simulink model "combined_models_v16"  (R2021a)
settings: Solver=VariableStepAuto  StartTime=0.0  StopTime=30  RelTol=1e-3
values from neighbouring files (symbols this model uses):
  r__s_st = r__s_stCG - r__t_tCG    [init_saildrone_dynamics_v5.m]    (also in moduleBasedModel_v7.m = cfg.r__s_st; systemVelocities.m = cfg.r__s_st)
  r__t_tAC = r__t_tCG    [init_saildrone_dynamics_v5.m]
  rho = 1025    [init_saildrone_dynamics_v5.m]    (also in moduleBasedModel_v7.m = cfg.rho; simplifiedModel_v8.m = cfg.rho)
  rho_air = 1.225    [init_saildrone_dynamics_v5.m]
undefined symbols (not defined in the file or in its folder): beta_V_w, cfg, delta_LOS, DiscIntNeverNeededParam, gamma_c, GWP, heading_controller_samplingtime, heading_rate_ref, K_b, K_d_heading, K_d_heading2, K_d_s, k_d_s, K_d_t, K_i_heading, K_i_heading2, K_i_s, k_i_s, K_i_t, K_p_heading, K_p_heading2, k_p_s, K_p_s, K_p_t, Ka_lin, keel, ObjectsPosition, omega_n_heading2, omega_n_s, q0, q_dot0, rudder, sail, sail_AOA_controller_samplingtime, sail_AOA_linearization_point, sail_AOA_saturation, sail_AOA_table, simulation_sampling_time, start_w_trans, tacking_minus, tacking_plus, tail, theta0, timeconstant_w, U_c, U_linearization_heading, U_w, U_w_step, v_current, v_wind, v_wind_unit, wn_ref_heading, wn_ref_t, xi0, zeta_ref_heading, zeta_ref_t
(part 1 of 3)
settings Model: Creator=jorge  LastModifiedBy=jorge

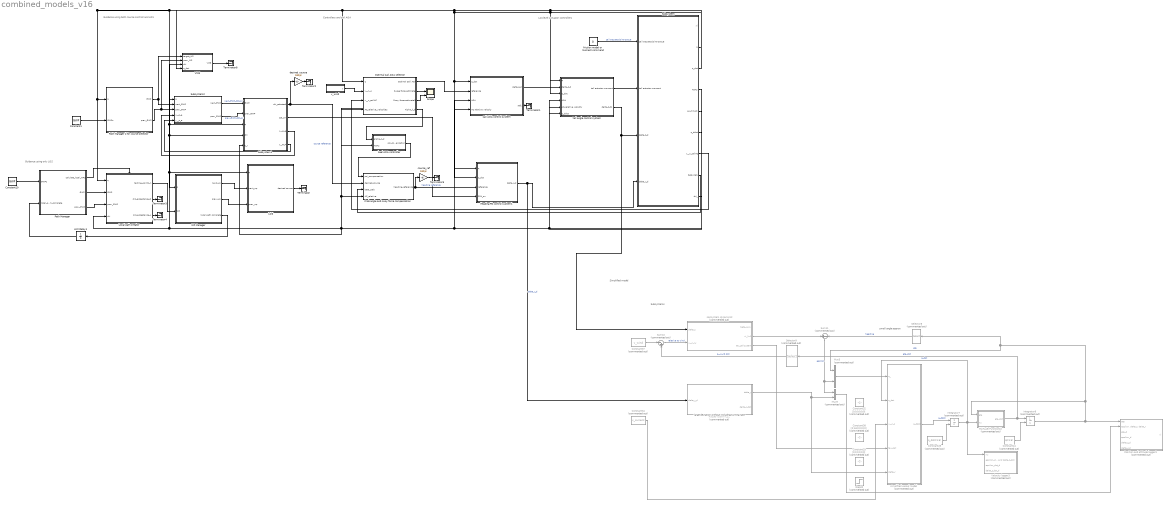
== system combined_models_v16 ==
  note: Guidance using only LOS
  note: Guidance using both course controll and LOS
  note: Controllers and sail AOA
  note: Lowlevel Actuator controllers
  note: Subsystems
  note: small angle approx
  note: large deviation without including turning rate
  note: Simplified model
  Constant1 : Constant  Value=GWP
  Constant10 : Constant  Value=GWP
  Constant24 : Constant  Commented=on  Value=q0(1:6)
  Constant25 : Constant  Commented=on  Value=q_dot0(1:6)
  Constant32 : Constant  Commented=on  Value=[0;0;0;0;0;0]
  Constant33 : Constant  Commented=on  Value=[0;0;0;0;0;0]
  Constant34 : Constant  Commented=on  Value=v_current
  Constant37 : Constant  Commented=on  Value=v_wind
  Constant38 : Constant  Commented=on  Value=[0;140;0;0;0;0]
  "Crab angle and sway force compensation " : MATLAB Function  TreatAsAtomicUnit=on
  Heading PD control system1 : Subsystem
  Integrator7 : Integrator  Commented=on  InitialConditionSource=external
  Integrator8 : Integrator  Commented=on  InitialConditionSource=external
  LOS : Subsystem
  Local path creator : Subsystem
  MATLAB Function10 : MATLAB Function  Commented=on  TreatAsAtomicUnit=on
  Mux3 : Mux  Commented=on  Inputs=2
  Mux9 : Mux  Commented=on  Inputs=3
  Optimal sail AOA selector : Subsystem
  Path Manager : Subsystem
  Path Manager 2 for course selector : Subsystem
  Position and attitude logger3 : Subsystem  Commented=on
  Rudder dyanmics2 : Subsystem  Commented=on
  Scope : Scope  NumInputPorts=2
  Selector8 : Selector  Commented=on  InputPortWidth=6  IndexOptions=Index vector (dialog)  Indices=[6]  OutputSizes=1
  Selector9 : Selector  Commented=on  InputPortWidth=6  IndexOptions=Index vector (dialog)  Indices="[1  2 3]"  OutputSizes=1
  Step20 : Step  Commented=on  After=-pi/4*1  SampleTime=0
  Subsystem : Subsystem
  Subsystem1 : Subsystem
  Subsystem2 : Subsystem
  Sum10 : Sum  Commented=on  Inputs=|-+
  Sum11 : Sum  Commented=on  Inputs=+-
  Terminator{,1..5,8} (7 alike) : Terminator
  Unit Delay1 : UnitDelay  SampleTime=-1  HasFrameUpgradeWarning=on
  VMG : MATLAB Function  TreatAsAtomicUnit=on
  Velocity logger3 : Subsystem  Commented=on
  WP Manager : Subsystem
  course_ref : Gain  Gain=180/pi
  desired_course : Gain  Gain=180/pi
  friction model or moment command : Constant  Value=0
  keel AOA controller : Subsystem
  sail AOA control system : Subsystem
  sailsystem dynamics2 : Subsystem  Commented=on
  simplified vessel model : MATLAB Function  Commented=on  TreatAsAtomicUnit=on
  tail angle control system : Subsystem
  v_wind : Subsystem
  wires:
  friction model or moment command/1 -> Subsystem/1(sail actuator/joint torque)  "sail actuator/joint torque"
  Subsystem/4(AOAs) -> tail angle control system/4(AOA), sail AOA control system/3(AOA), keel AOA controller/2(AOAs)
  Subsystem/3(q_dot) -> Heading PD control system1/2(q_dot), sail AOA control system/1(q_dot), VMG/4(q_dot), tail angle control system/3(q_dot)
  Subsystem/6(q_ddot) -> tail angle control system/6(q_ddot)
  tail angle control system/1(tail actuator moment) -> Subsystem/2(tail actuator moment)
  Subsystem/5(U_r_linkAC) -> tail angle control system/5(AC_relative velocity), sail AOA control system/4(AC relative velocity), Optimal sail AOA selector/4(AC_relative_velocities), "Crab angle and sway force compensation "/4(AC_relative), Subsystem1/5(U_r)
  Subsystem/7(v__n_sailAC) -> Optimal sail AOA selector/3(v__n_sailAC)
  Optimal sail AOA selector/2(Surge force estimate) -> Scope/1
  Optimal sail AOA selector/3(Sway force estimate1) -> Scope/2
  Subsystem/2(q) -> Heading PD control system1/1(q), Path Manager 2 for course selector/1(q), Local path creator/1(q), Subsystem2/1(q), Subsystem1/3(q), WP Manager/1(q), LOS/1(q), Optimal sail AOA selector/1(q), tail angle control system/1(q)
  sail AOA control system/2(ref1) -> Terminator1/1
  Constant24/1 -> Integrator8/2
  sailsystem dynamics2/3(tau_sailsystem) -> simplified vessel model/4(tau_sail)
  Constant25/1 -> Integrator7/2
  Rudder dyanmics2/1(delta_r) -> simplified vessel model/5(delta_r), Mux9/3
  Sum11/1 -> Mux3/2, Mux9/1  "epsilon"
  Integrator8/1 -> Selector8/1, Mux3/1, MATLAB Function10/1(eta), Position and attitude logger3/1(eta)  "eta"
  Constant34/1 -> simplified vessel model/3(v__n_c)
  Heading PD control system1/1(delta_r_d) -> Rudder dyanmics2/1(delta_r_d), Subsystem/4(delta_r_d)  "delta_r_d"
  Mux9/1 -> Position and attitude logger3/2("epsilon, delta_t, delta_r")
  Selector9/1 -> Sum10/2  "p__n_nb dot"
  simplified vessel model/1(q_ddot) -> Integrator7/1  "q_ddot"
  Sum10/1 -> sailsystem dynamics2/2(v__n_rw)  "relative to wind"
  Integrator7/1 -> Velocity logger3/1(nu), MATLAB Function10/2(nu), simplified vessel model/2(q_dot)  "q_dot"
  Selector8/1 -> Sum11/2  "heading"
  Constant37/1 -> Sum10/1
  sailsystem dynamics2/2(xi_lin1) -> Sum11/1
  MATLAB Function10/1(eta_dot) -> Selector9/1, Integrator8/1  "eta_dot"
  Mux3/1 -> simplified vessel model/1(q_)
  Optimal sail AOA selector/4(Alpha_k_d) -> keel AOA controller/1(alpha_k_d)
  Subsystem1/1(chi_selected) -> "Crab angle and sway force compensation "/2(desired_course), desired_course/1  "course reference"
  Subsystem/8(beta crab) -> "Crab angle and sway force compensation "/3(beta_crab)
  desired_course/1 -> Terminator2/1
  WP Manager/1(next_wp) -> LOS/2(next_wp)
  WP Manager/2(prev_wp) -> LOS/3(prev_wp)
  keel AOA controller/1(psi_compensation) -> "Crab angle and sway force compensation "/1(psi_compensation)
  WP Manager/3(local path complete) -> Unit Delay1/1
  Local path creator/2(circ_acceptance_R) -> Terminator3/1
  Local path creator/1(tacking_points_n) -> WP Manager/2(WP)
  Local path creator/3(circ_acceptance_L) -> Terminator4/1
  Subsystem/9(chi_) -> VMG/3(chi), Subsystem1/4(chi), Local path creator/4(chi)
  Path Manager/1(calulate_local_WPs) -> Local path creator/Enable
  Path Manager/3(prev_GWP) -> Local path creator/3(prev_GWP)
  Path Manager/2(GWP) -> Local path creator/2(GWP)
  Constant10/1 -> Path Manager/1(GWPs)
  Unit Delay1/1 -> Path Manager/2(local_path_complete)
  Constant1/1 -> Path Manager 2 for course selector/2(GWPs)
  Subsystem1/2(ssa_on) -> Heading PD control system1/4(SSA_on)
  Subsystem1/3(x__p_e) -> Subsystem2/4(x__p_e)
  Subsystem1/4(y__e_p) -> Subsystem2/5(y__p_e)
  Path Manager 2 for course selector/1(GWP) -> VMG/1(target_WP), Subsystem2/2("next_GWP ")
  Path Manager 2 for course selector/2(prev_GWP) -> Subsystem2/3("prev_GWP "), VMG/2(prev_WP)
  Subsystem2/2(prev_GWP) -> Subsystem1/2(prev_GWP)  "prev_GWP_COLAV"
  Subsystem2/1(next_GWP) -> Subsystem1/1(GWP)  "next_GWP_COLAV"
  course_ref/1 -> Terminator5/1
  "Crab angle and sway force compensation "/1(heading_reference) -> course_ref/1, Heading PD control system1/3(reference)  "heading reference"
  VMG/1(VMG) -> Terminator8/1
  tail angle control system/2(delta_t_d1) -> sailsystem dynamics2/1(delta_t), Subsystem/3(delta_t_d)
  Optimal sail AOA selector/1(Optimal Sail AOA) -> sail AOA control system/2(reference)
  sail AOA control system/1(delta_t_d) -> tail angle control system/2(delta_t_d)
  v_wind/1(y) -> Optimal sail AOA selector/2(v__n_w)
  LOS/1(desired course) -> Terminator/1

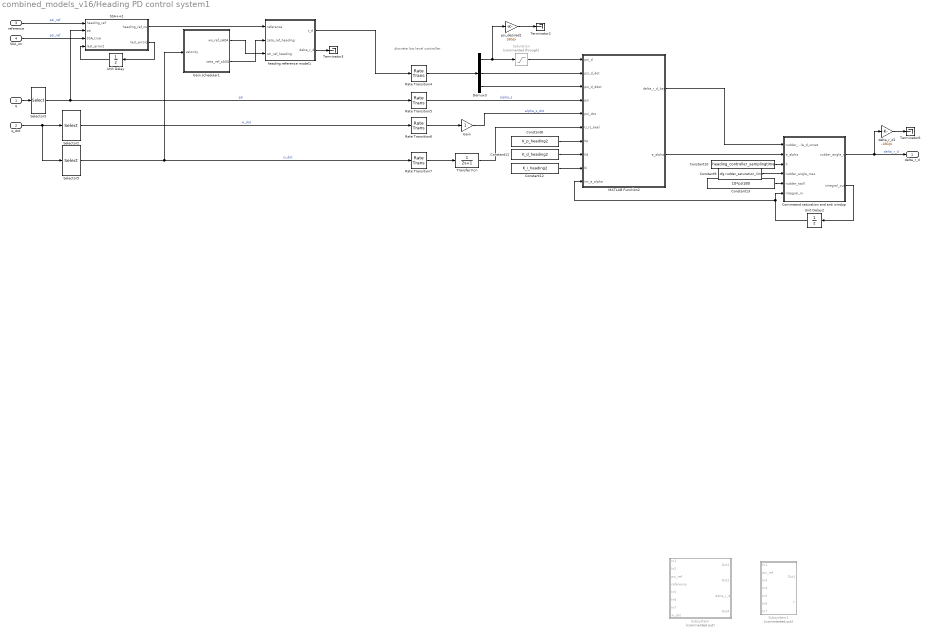
== system combined_models_v16/Heading PD control system1 ==
  note: discrete low
      | level controller
  q : Inport
  q_dot : Inport  Port=2
  reference : Inport  Port=3
  SSA_on : Inport  Port=4
  Commeand saturation and anti windup : MATLAB Function  TreatAsAtomicUnit=on
  Constant10 : Constant  Value=heading_controller_samplingtime
  Constant11 : Constant  Value=K_d_heading2
  Constant12 : Constant  Value=K_i_heading2
  Constant13 : Constant  Value=10*pi/180
  Constant8 : Constant  Value=K_p_heading2
  Constant9 : Constant  Value=cfg.rudder_saturation_limit
  Demux3 : Demux  Outputs=3
  Gain : Gain
  Gain scheduler1 : Subsystem
  MATLAB Function2 : MATLAB Function  TreatAsAtomicUnit=on
  Rate Transition{4..7} (4 alike) : RateTransition  OutPortSampleTime=heading_controller_samplingtime
  SSA++2 : MATLAB Function  TreatAsAtomicUnit=on
  Saturation : Saturate  Commented=through  UpperLimit=sail_AOA_saturation  LowerLimit=-sail_AOA_saturation
  Selector2 : Selector  InputPortWidth=8  IndexOptions=Index vector (dialog)  Indices=[6]  OutputSizes=1
  Selector3 : Selector  InputPortWidth=9  IndexOptions=Index vector (dialog)  Indices=[6]  OutputSizes=1
  Selector5 : Selector  InputPortWidth=8  IndexOptions=Index vector (dialog)  Indices=[1]  OutputSizes=1
  Subsystem : Subsystem  Commented=on
  Subsystem1 : Subsystem  Commented=on
  Terminator2 : Terminator
  Terminator3 : Terminator
  Terminator6 : Terminator
  Transfer Fcn : TransferFcn  Denominator=[2 1]
  Unit Delay : UnitDelay  SampleTime=-1  HasFrameUpgradeWarning=on
  Unit Delay2 : UnitDelay  SampleTime=heading_controller_samplingtime  HasFrameUpgradeWarning=on
  delta_r_d1 : Gain  Gain=-180/pi
  heading reference model1 : Subsystem
  psi_desired2 : Gain  Gain=180/pi
  delta_r_d : Outport
  wires:
  reference/1 -> SSA++2/1(heading_ref)  "psi_ref"
  q_dot/1 -> Selector5/1, Selector2/1
  q/1 -> Selector3/1
  SSA++2/1(heading_ref_cor) -> heading reference model1/1(reference)
  SSA++2/2(last_error2) -> Unit Delay/1
  Unit Delay/1 -> SSA++2/4("last_error2 ")
  SSA_on/1 -> SSA++2/3(SSA_true)  "psi_ref"
  Demux3/2 -> MATLAB Function2/2(psi_d_dot)
  Unit Delay2/1 -> Commeand saturation and anti windup/6(integral_in), MATLAB Function2/10(int_e_alpha)
  Constant12/1 -> MATLAB Function2/9(Ki)
  MATLAB Function2/1(delta_r_d_bar) -> Commeand saturation and anti windup/1(rudder_angle_d_unsat)
  Constant11/1 -> MATLAB Function2/8(Kd)
  Rate Transition7/1 -> Transfer Fcn/1
  Gain/1 -> MATLAB Function2/5(psi_dot)  "alpha_s_dot"
  Commeand saturation and anti windup/2(integral_out) -> Unit Delay2/1
  Constant10/1 -> Commeand saturation and anti windup/3(h)
  Selector2/1 -> Rate Transition6/1  "xi_dot"
  Rate Transition5/1 -> MATLAB Function2/4(psi)  "alpha_s"
  Rate Transition6/1 -> Gain/1
  Demux3/3 -> MATLAB Function2/3(psi_d_ddot)
  Constant9/1 -> Commeand saturation and anti windup/4(rudder_angle_max)
  Selector3/1 -> SSA++2/2(psi), Rate Transition5/1  "psi"
  Rate Transition4/1 -> Demux3/1
  Constant8/1 -> MATLAB Function2/7(Kp)
  Demux3/1 -> Saturation/1, psi_desired2/1
  MATLAB Function2/2(e_alpha) -> Commeand saturation and anti windup/2(e_alpha)
  Saturation/1 -> MATLAB Function2/1(psi_d)
  Constant13/1 -> Commeand saturation and anti windup/5(rudder_stall)
  Transfer Fcn/1 -> MATLAB Function2/6(U_rc_keel)
  Selector5/1 -> Rate Transition7/1, Gain scheduler1/1(velocity)  "xi_dot"
  Gain scheduler1/1(wn_ref_sAOA) -> heading reference model1/3(wn_ref_heading)
  Gain scheduler1/2(zeta_ref_sAOA) -> heading reference model1/2(zeta_ref_heading)
  heading reference model1/1(x_d) -> Rate Transition4/1
  psi_desired2/1 -> Terminator2/1
  delta_r_d1/1 -> Terminator6/1
  Commeand saturation and anti windup/1(rudder_angle_d) -> delta_r_d1/1, delta_r_d/1  "delta_r_d"
  heading reference model1/2(delta_r_d) -> Terminator3/1

== system combined_models_v16/LOS ==
  q : Inport
  next_wp : Inport  Port=2
  prev_wp : Inport  Port=3
  Constant3 : Constant  Value=delta_LOS
  Descrete : RateTransition  OutPortSampleTime=LOS_samplingtime
  MATLAB Function2 : MATLAB Function  TreatAsAtomicUnit=on
  desired course : Outport
  wires:
  MATLAB Function2/1(chi_d) -> desired course/1  "desired course"
  Constant3/1 -> MATLAB Function2/3(delta)
  Descrete/1 -> MATLAB Function2/4(q)
  prev_wp/1 -> MATLAB Function2/2(prev_wp)
  next_wp/1 -> MATLAB Function2/1(next_wp)
  q/1 -> Descrete/1

== system combined_models_v16/Local path creator ==
  q : Inport
  GWP : Inport  Port=2
  prev_GWP : Inport  Port=3
  chi : Inport  Port=4
  Enable : EnablePort
  Constant1 : Constant  Value=gamma_c
  Constant10 : Constant  Value=beta_V_w
  Constant11 : Constant  Value=U_w
  Constant12 : Constant  Value=tacking_minus
  Constant13 : Constant  Value=tacking_plus
  Constant14 : Constant  Value=U_c
  Constant9 : Constant  Value=0
  Display : Display
  MATLAB Function3 : MATLAB Function  TreatAsAtomicUnit=on
  Sum : Sum  Inputs=|++
  Sum1 : Sum  Inputs=++|
  init size : Constant  Commented=on  Value=[0;0]
  init size1 : Constant  Commented=on  Value=[0;0]
  tacking_points_n : Outport  InitialOutput=[zeros(2,100)]
  circ_acceptance_R : Outport  Port=2
  circ_acceptance_L : Outport  Port=3
  wires:
  MATLAB Function3/2(circ_acceptance_R) -> circ_acceptance_R/1
  MATLAB Function3/1(tacking_points_n) -> Display/1, tacking_points_n/1
  MATLAB Function3/3(circ_acceptance_L) -> circ_acceptance_L/1
  q/1 -> MATLAB Function3/3(q)
  Sum/1 -> MATLAB Function3/2(prev_WP)
  Sum1/1 -> MATLAB Function3/1(target_WP)
  Constant1/1 -> MATLAB Function3/5(beta_c)
  Constant9/1 -> MATLAB Function3/6(U_c)
  Constant10/1 -> MATLAB Function3/7(beta_w)
  Constant11/1 -> MATLAB Function3/8(U_w)
  Constant12/1 -> MATLAB Function3/9(tacking_minus)
  Constant13/1 -> MATLAB Function3/10(tacking_plus)
  chi/1 -> MATLAB Function3/4(chi)
  init size/1 -> Sum/2
  prev_GWP/1 -> Sum/1
  GWP/1 -> Sum1/2
  init size1/1 -> Sum1/1

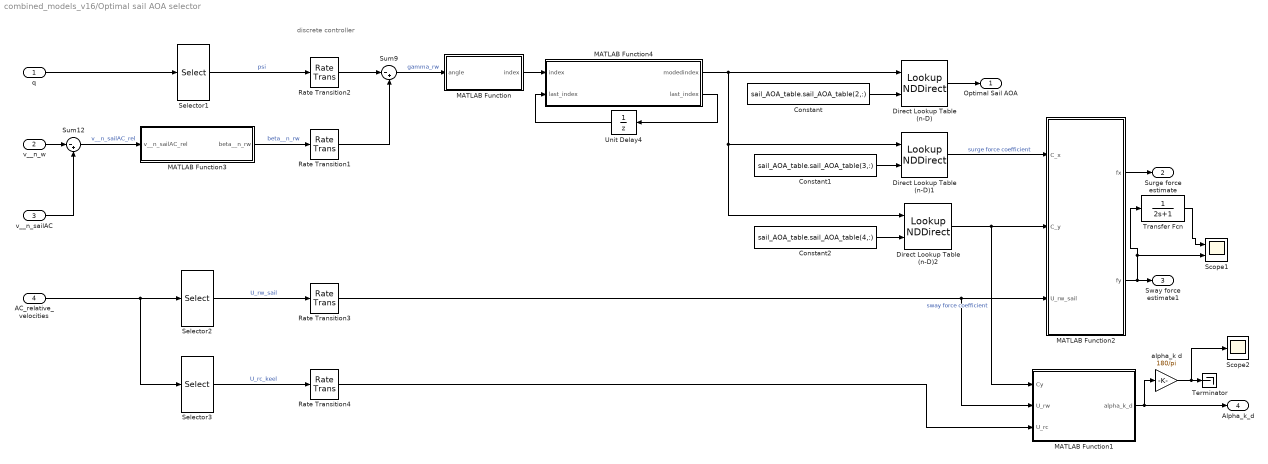
== system combined_models_v16/Optimal sail AOA selector ==
  note: discrete
      | controller
  q : Inport
  v__n_w : Inport  Port=2
  v__n_sailAC : Inport  Port=3
  AC_relative_velocities : Inport  Port=4
  Constant : Constant  Value=sail_AOA_table.sail_AOA_table(2,:)
  Constant1 : Constant  Value=sail_AOA_table.sail_AOA_table(3,:)
  Constant2 : Constant  Value=sail_AOA_table.sail_AOA_table(4,:)
  Direct Lookup Table (n-D) : LookupNDDirect  NumberOfTableDimensions=1  TableIsInput=on
  Direct Lookup Table (n-D)1 : LookupNDDirect  NumberOfTableDimensions=1  TableIsInput=on
  Direct Lookup Table (n-D)2 : LookupNDDirect  NumberOfTableDimensions=1  TableIsInput=on
  MATLAB Function : MATLAB Function  TreatAsAtomicUnit=on
  MATLAB Function1 : MATLAB Function  TreatAsAtomicUnit=on
  MATLAB Function2 : MATLAB Function  TreatAsAtomicUnit=on
  MATLAB Function3 : MATLAB Function  TreatAsAtomicUnit=on
  MATLAB Function4 : MATLAB Function  TreatAsAtomicUnit=on
  Rate Transition{1..4} (4 alike) : RateTransition  OutPortSampleTime=sail_AOA_lookup_samplingtime
  Scope1 : Scope  NumInputPorts=2
  Scope2 : Scope
  Selector1 : Selector  InputPortWidth=9  IndexOptions=Index vector (dialog)  Indices=[6]  OutputSizes=1
  Selector2 : Selector  InputPortWidth=4  IndexOptions=Index vector (dialog)  Indices=[2]  OutputSizes=1
  Selector3 : Selector  InputPortWidth=4  IndexOptions=Index vector (dialog)  Indices=[1]  OutputSizes=1
  Sum12 : Sum  Inputs=|-+
  Sum9 : Sum  Inputs=|-+
  Terminator : Terminator
  Transfer Fcn : TransferFcn  Denominator=[2 1]
  Unit Delay4 : UnitDelay  InitialCondition=-999  SampleTime=-1  HasFrameUpgradeWarning=on
  alpha_k d : Gain  Gain=180/pi
  Optimal Sail AOA : Outport
  Surge force estimate : Outport  Port=2
  Sway force estimate1 : Outport  Port=3
  Alpha_k_d : Outport  Port=4
  wires:
  Rate Transition1/1 -> Sum9/2
  MATLAB Function3/1(beta__n_rw) -> Rate Transition1/1  "beta__n_rw"
  Constant/1 -> Direct Lookup Table (n-D)/2
  MATLAB Function4/1(modedindex) -> Direct Lookup Table (n-D)/1, Direct Lookup Table (n-D)2/1, Direct Lookup Table (n-D)1/1
  Sum12/1 -> MATLAB Function3/1(v__n_sailAC_rel)  "v__n_sailAC_rel"
  Rate Transition2/1 -> Sum9/1
  Selector1/1 -> Rate Transition2/1  "psi"
  v__n_w/1 -> Sum12/1
  q/1 -> Selector1/1
  v__n_sailAC/1 -> Sum12/2
  Constant1/1 -> Direct Lookup Table (n-D)1/2
  Direct Lookup Table (n-D)1/1 -> MATLAB Function2/1(C_x)  "surge force coefficient"
  Constant2/1 -> Direct Lookup Table (n-D)2/2
  Direct Lookup Table (n-D)2/1 -> MATLAB Function2/2(C_y), MATLAB Function1/1(Cy)  "sway force coefficient"
  AC_relative_velocities/1 -> Selector3/1, Selector2/1
  Selector2/1 -> Rate Transition3/1  "U_rw_sail"
  MATLAB Function2/1(fx) -> Surge force estimate/1
  MATLAB Function2/2(fy) -> Transfer Fcn/1, Scope1/2, Sway force estimate1/1
  Rate Transition3/1 -> MATLAB Function1/2(U_rw), MATLAB Function2/3(U_rw_sail)
  MATLAB Function4/2(last_index) -> Unit Delay4/1
  Unit Delay4/1 -> MATLAB Function4/2("last_index ")
  MATLAB Function/1(index) -> MATLAB Function4/1(index)
  Transfer Fcn/1 -> Scope1/1
  Selector3/1 -> Rate Transition4/1  "U_rc_keel"
  Rate Transition4/1 -> MATLAB Function1/3(U_rc)
  MATLAB Function1/1(alpha_k_d) -> Alpha_k_d/1, alpha_k d/1
  alpha_k d/1 -> Scope2/1, Terminator/1
  Direct Lookup Table (n-D)/1 -> Optimal Sail AOA/1
  Sum9/1 -> MATLAB Function/1(angle)  "gamma_rw"

== system combined_models_v16/Path Manager ==
  GWPs : Inport
  local_path_complete : Inport  Port=2
  Display1 : Display
  Display2 : Display
  Path Manager : MATLAB Function  TreatAsAtomicUnit=on
  Sum1 : Sum  Inputs=|++
  Sum2 : Sum  Inputs=++|
  Sum3 : Sum  Inputs=++|
  Unit Delay : UnitDelay  InitialCondition=1  SampleTime=-1  HasFrameUpgradeWarning=on
  init calculations : Step  Time=0.1  Before=1  After=0  SampleTime=0
  init size1 : Constant  Value=[0;0]
  init size2 : Constant  Value=[0;0]
  calulate_local_WPs : Outport
  GWP : Outport  Port=2
  prev_GWP : Outport  Port=3
  wires:
  Path Manager/4(GWP_index) -> Unit Delay/1
  local_path_complete/1 -> Path Manager/2(local_path_complete)
  Path Manager/3(calulate_local_WPs) -> Sum1/1
  Sum2/1 -> GWP/1, Display2/1
  Unit Delay/1 -> Path Manager/3("GWP_index ")
  Sum3/1 -> Display1/1, prev_GWP/1
  GWPs/1 -> Path Manager/1(GWPs)
  init calculations/1 -> Sum1/2
  Sum1/1 -> calulate_local_WPs/1
  init size1/1 -> Sum2/1
  Path Manager/1(GWP) -> Sum2/2
  Path Manager/2(prev_GWP) -> Sum3/2
  init size2/1 -> Sum3/1

== system combined_models_v16/Path Manager 2 for course selector ==
  q : Inport
  GWPs : Inport  Port=2
  Display1 : Display
  Display2 : Display
  Path Manager : MATLAB Function  TreatAsAtomicUnit=on
  Sum2 : Sum  Inputs=++|
  Sum3 : Sum  Inputs=++|
  Unit Delay : UnitDelay  InitialCondition=1  SampleTime=-1  HasFrameUpgradeWarning=on
  init size1 : Constant  Value=[0;0]
  init size2 : Constant  Value=[0;0]
  GWP : Outport
  prev_GWP : Outport  Port=2
  wires:
  Path Manager/3(GWP_index) -> Unit Delay/1
  q/1 -> Path Manager/1(q)
  Sum2/1 -> GWP/1, Display2/1
  Unit Delay/1 -> Path Manager/3("GWP_index ")
  Sum3/1 -> Display1/1, prev_GWP/1
  GWPs/1 -> Path Manager/2(GWPs)
  init size1/1 -> Sum2/1
  Path Manager/1(GWP) -> Sum2/2
  Path Manager/2(prev_GWP) -> Sum3/2
  init size2/1 -> Sum3/1

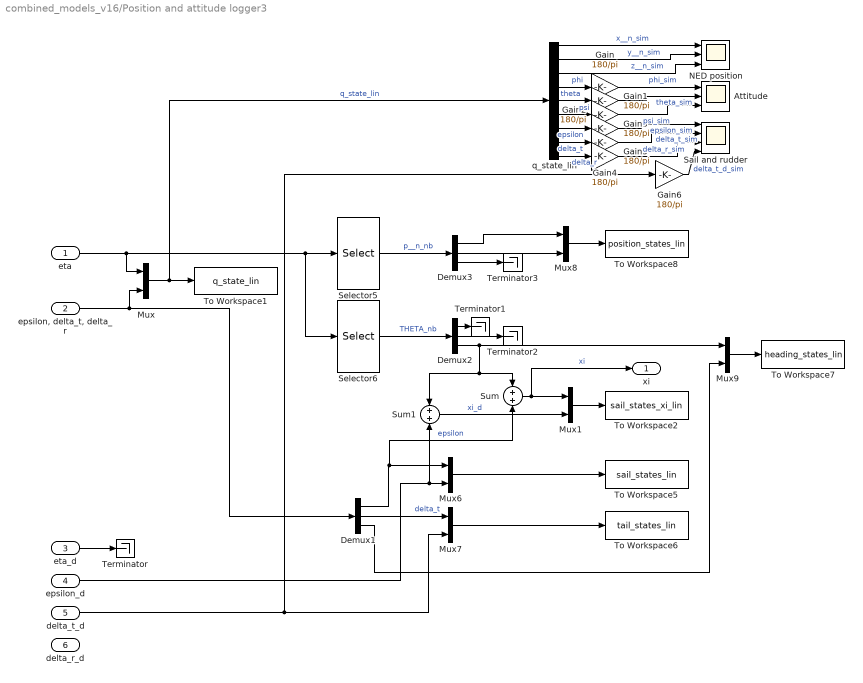
== system combined_models_v16/Position and attitude logger3 ==
  eta : Inport
  "epsilon, delta_t, delta_r" : Inport  Port=2
  eta_d : Inport  Port=3
  epsilon_d : Inport  Port=4
  delta_t_d : Inport  Port=5
  delta_r_d : Inport  Port=6
  Attitude : Scope  NumInputPorts=3
  Demux1 : Demux  Outputs=3
  Demux2 : Demux  Outputs=3
  Demux3 : Demux  Outputs=3
  Gain{,1..6} (7 alike) : Gain  Gain=180/pi
  Mux{,1,6..9} (6 alike) : Mux  Inputs=2
  NED position : Scope  NumInputPorts=3
  Sail and rudder : Scope  NumInputPorts=4
  Selector5 : Selector  InputPortWidth=6  IndexOptions=Index vector (dialog)  Indices=[1 2 3]  OutputSizes=1
  Selector6 : Selector  InputPortWidth=6  IndexOptions=Index vector (dialog)  Indices=[4 5 6]  OutputSizes=1
  Sum : Sum  Inputs=+|+
  Sum1 : Sum  Inputs=+|+
  Terminator{,1..3} (4 alike) : Terminator
  To Workspace1 : ToWorkspace  VariableName=q_state_lin  SampleTime=-1
  To Workspace2 : ToWorkspace  VariableName=sail_states_xi_lin  SampleTime=simulation_sampling_time
  To Workspace5 : ToWorkspace  VariableName=sail_states_lin  SampleTime=simulation_sampling_time
  To Workspace6 : ToWorkspace  VariableName=tail_states_lin  SampleTime=simulation_sampling_time
  To Workspace7 : ToWorkspace  VariableName=heading_states_lin  SampleTime=simulation_sampling_time
  To Workspace8 : ToWorkspace  VariableName=position_states_lin  SampleTime=simulation_sampling_time
  q_state_lin : Demux  Outputs=9
  xi : Outport
  wires:
  Demux2/3 -> Sum1/1, Sum/1, Mux9/1
  eta/1 -> Mux/1, Selector6/1, Selector5/1
  Demux3/1 -> Mux8/1
  Selector5/1 -> Demux3/1  "p__n_nb"
  Mux8/1 -> To Workspace8/1
  Mux9/1 -> To Workspace7/1
  Demux1/2 -> Mux7/1  "delta_t"
  Demux3/2 -> Mux8/2
  Mux6/1 -> To Workspace5/1
  Selector6/1 -> Demux2/1  "THETA_nb"
  Demux1/1 -> Sum/2, Mux6/1  "epsilon"
  Mux7/1 -> To Workspace6/1
  "epsilon, delta_t, delta_r"/1 -> Mux/2, Demux1/1
  delta_t_d/1 -> Gain6/1, Mux7/2
  epsilon_d/1 -> Mux6/2, Sum1/2
  eta_d/1 -> Terminator/1
  Demux2/2 -> Terminator2/1
  Demux2/1 -> Terminator1/1
  Demux3/3 -> Terminator3/1
  Mux/1 -> q_state_lin/1, To Workspace1/1  "q_state_lin"
  Demux1/3 -> Mux9/2
  Sum/1 -> xi/1, Mux1/1  "xi"
  Sum1/1 -> Mux1/2  "xi_d"
  Mux1/1 -> To Workspace2/1
  q_state_lin/6 -> Gain2/1  "psi"
  q_state_lin/7 -> Gain3/1  "epsilon"
  q_state_lin/5 -> Gain1/1  "theta"
  Gain4/1 -> Sail and rudder/2  "delta_t_sim"
  Gain/1 -> Attitude/1  "phi_sim"
  Gain5/1 -> Sail and rudder/3  "delta_r_sim"
  Gain2/1 -> Attitude/3  "psi_sim"
  Gain3/1 -> Sail and rudder/1  "epsilon_sim"
  q_state_lin/8 -> Gain4/1  "delta_t"
  Gain1/1 -> Attitude/2  "theta_sim"
  q_state_lin/4 -> Gain/1  "phi"
  q_state_lin/1 -> NED position/1  "x__n_sim"
  q_state_lin/9 -> Gain5/1  "delta_r"
  q_state_lin/3 -> NED position/3  "z__n_sim"
  q_state_lin/2 -> NED position/2  "y__n_sim"
  Gain6/1 -> Sail and rudder/4  "delta_t_d_sim"

== system combined_models_v16/Rudder dyanmics2 ==
  delta_r_d : Inport
  1st order rudder dynamics1 : Subsystem
  delta_r1 : Constant  Value=q0(9)
  delta_r : Outport
  delta_r_dot : Outport  Port=2
  wires:
  1st order rudder dynamics1/1(delta_r_dot) -> delta_r_dot/1
  1st order rudder dynamics1/2(delta_r) -> delta_r/1  "delta_r"
  delta_r1/1 -> 1st order rudder dynamics1/1(delta_r0)
  delta_r_d/1 -> 1st order rudder dynamics1/2(delta_r_d)

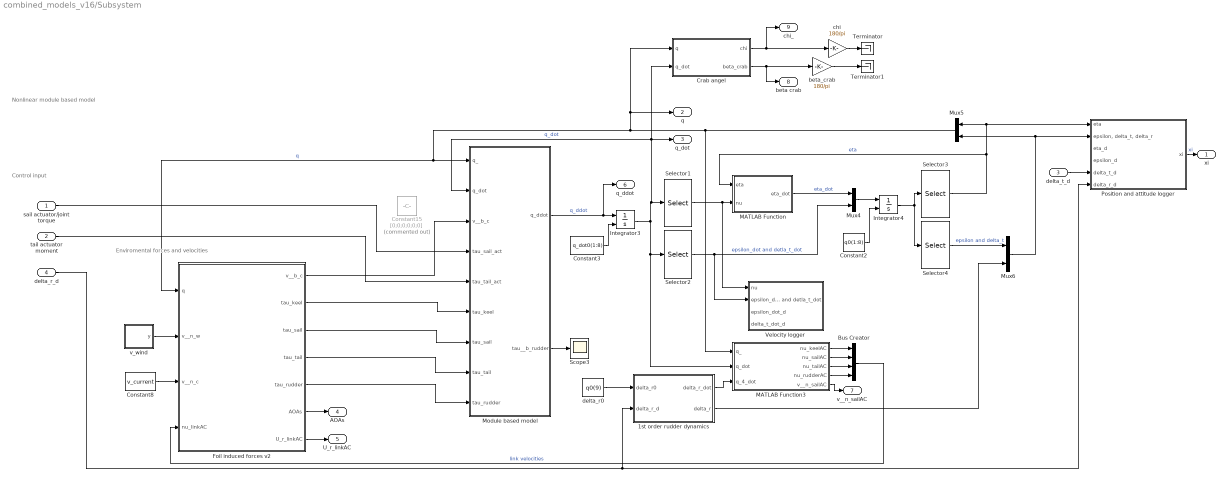
== system combined_models_v16/Subsystem ==
  note: Control input
  note: Enviromental forces and velocities
  note: Nonlinear module based model
  sail actuator/joint torque : Inport
  tail actuator moment : Inport  Port=2
  delta_t_d : Inport  Port=3
  delta_r_d : Inport  Port=4
  1st order rudder dynamics : Subsystem
  Bus Creator : BusCreator  Inputs=4
  Constant15 : Constant  Commented=on  Value=[0;0;0;0;0;0]
  Constant2 : Constant  Value=q0(1:8)
  Constant3 : Constant  Value=q_dot0(1:8)
  Constant8 : Constant  Value=v_current
  Crab angel : MATLAB Function  TreatAsAtomicUnit=on
  Foil induced forces v2 : Subsystem
  Integrator3 : Integrator  InitialConditionSource=external
  Integrator4 : Integrator  InitialConditionSource=external
  MATLAB Function : MATLAB Function  TreatAsAtomicUnit=on
  MATLAB Function3 : MATLAB Function  TreatAsAtomicUnit=on
  Module based model : MATLAB Function  TreatAsAtomicUnit=on
  Mux4 : Mux  Inputs=2
  Mux5 : Mux  Inputs=2
  Mux6 : Mux  Inputs=2
  Position and attitude logger : Subsystem
  Scope3 : Scope
  Selector1 : Selector  InputPortWidth=8  IndexOptions=Index vector (dialog)  Indices=[1 2 3 4 5 6]  OutputSizes=1
  Selector2 : Selector  InputPortWidth=8  IndexOptions=Index vector (dialog)  Indices=[7 8]  OutputSizes=1
  Selector3 : Selector  InputPortWidth=8  IndexOptions=Index vector (dialog)  Indices=[1 2 3 4 5 6]  OutputSizes=1
  Selector4 : Selector  InputPortWidth=8  IndexOptions=Index vector (dialog)  Indices=[7 8]  OutputSizes=1
  Terminator : Terminator
  Terminator1 : Terminator
  Velocity logger : Subsystem
  beta_crab : Gain  Gain=180/pi
  chi : Gain  Gain=180/pi
  delta_r0 : Constant  Value=q0(9)
  v_wind : Subsystem
  xi : Outport
  q : Outport  Port=2
  q_dot : Outport  Port=3
  AOAs : Outport  Port=4
  U_r_linkAC : Outport  Port=5
  q_ddot : Outport  Port=6
  v__n_sailAC : Outport  Port=7
  beta crab : Outport  Port=8
  chi_ : Outport  Port=9
  wires:
  MATLAB Function3/3(nu_tailAC) -> Bus Creator/3
  Integrator3/1 -> Selector1/1, Crab angel/2(q_dot), Module based model/2(q_dot), q_dot/1, MATLAB Function3/2(q_dot), Selector2/1  "q_dot"
  MATLAB Function/1(eta_dot) -> Mux4/1  "eta_dot"
  Constant2/1 -> Integrator4/2
  Selector1/1 -> Velocity logger/1(nu), MATLAB Function/2(nu)
  delta_r_d/1 -> 1st order rudder dynamics/2(delta_r_d), Position and attitude logger/6(delta_r_d)
  Selector3/1 -> Mux5/1, Position and attitude logger/1(eta), MATLAB Function/1(eta)  "eta"
  Mux5/1 -> Foil induced forces v2/1(q), Module based model/1(q_), q/1, Crab angel/1(q), MATLAB Function3/1(q_)  "q"
  Foil induced forces v2/2(tau_keel) -> Module based model/6(tau_keel)
  delta_t_d/1 -> Position and attitude logger/5(delta_t_d)
  Selector2/1 -> Mux4/2, Velocity logger/2(epsilon_dot and detla_t_dot)  "epsilon_dot and detla_t_dot"
  MATLAB Function3/2(nu_sailAC) -> Bus Creator/2
  Mux6/1 -> Position and attitude logger/2("epsilon, delta_t, delta_r"), Mux5/2
  Mux4/1 -> Integrator4/1
  Integrator4/1 -> Selector3/1, Selector4/1
  delta_r0/1 -> 1st order rudder dynamics/1(delta_r0)
  Foil induced forces v2/1(v__b_c) -> Module based model/3(v__b_c)
  Selector4/1 -> Mux6/1  "epsilon and delta_t"
  MATLAB Function3/1(nu_keelAC) -> Bus Creator/1
  Bus Creator/1 -> Foil induced forces v2/4(nu_linkAC)  "link velocities"
  MATLAB Function3/4(nu_rudderAC) -> Bus Creator/4
  Foil induced forces v2/5(tau_rudder) -> Module based model/9(tau_rudder)
  1st order rudder dynamics/2(delta_r) -> Mux6/2
  Constant8/1 -> Foil induced forces v2/3(v__n_c)
  Module based model/2(tau__b_rudder) -> Scope3/1
  Module based model/1(q_ddot) -> q_ddot/1, Integrator3/1  "q_ddot"
  1st order rudder dynamics/1(delta_r_dot) -> MATLAB Function3/3(q_4_dot)
  tail actuator moment/1 -> Module based model/5(tau_tail_act)
  Foil induced forces v2/3(tau_sail) -> Module based model/7(tau_sail)
  Position and attitude logger/1(xi) -> xi/1  "xi"
  Constant3/1 -> Integrator3/2
  sail actuator/joint torque/1 -> Module based model/4(tau_sail_act)
  Foil induced forces v2/6(AOAs) -> AOAs/1
  Foil induced forces v2/7(U_r_linkAC) -> U_r_linkAC/1
  Foil induced forces v2/4(tau_tail) -> Module based model/8(tau_tail)
  MATLAB Function3/5(v__n_sailAC) -> v__n_sailAC/1
  Crab angel/1(chi) -> chi/1, chi_/1
  beta_crab/1 -> Terminator1/1
  chi/1 -> Terminator/1
  Crab angel/2(beta_crab) -> beta_crab/1, beta crab/1
  v_wind/1(y) -> Foil induced forces v2/2(v__n_w)

== system combined_models_v16/Subsystem1 ==
  GWP : Inport
  prev_GWP : Inport  Port=2
  q : Inport  Port=3
  chi : Inport  Port=4
  U_r : Inport  Port=5
  Constant1 : Constant  Value=gamma_c
  Constant10 : Constant  Value=beta_V_w
  Constant11 : Constant  Commented=on  Value=U_w
  Constant12 : Constant  Value=tacking_minus
  Constant13 : Constant  Value=tacking_plus
  Constant2 : Constant  Value=delta_LOS
  Constant9 : Constant  Value=U_c
  MATLAB Function : MATLAB Function  TreatAsAtomicUnit=on
  Selector : Selector  InputPortWidth=4  IndexOptions=Index vector (dialog)  Indices=[1]  OutputSizes=1
  Terminator1 : Terminator
  U_w : Subsystem
  Unit Delay : UnitDelay  SampleTime=-1  HasFrameUpgradeWarning=on
  Unit Delay1 : UnitDelay  InitialCondition=theta0  SampleTime=-1  HasFrameUpgradeWarning=on
  Unit Delay2 : UnitDelay  SampleTime=-1  HasFrameUpgradeWarning=on
  Unit Delay3 : UnitDelay  SampleTime=-1  HasFrameUpgradeWarning=on
  Unit Delay4 : UnitDelay  InitialCondition=[0;0]  SampleTime=-1  HasFrameUpgradeWarning=on
  Unit Delay5 : UnitDelay  InitialCondition=NaN(2,1)  SampleTime=-1  HasFrameUpgradeWarning=on
  Unit Delay6 : UnitDelay  InitialCondition=1  SampleTime=-1  HasFrameUpgradeWarning=on
  Unit Delay7 : UnitDelay  InitialCondition=-1  SampleTime=-1  HasFrameUpgradeWarning=on
  chi_selected : Outport
  ssa_on : Outport  Port=2
  x__p_e : Outport  Port=3
  y__e_p : Outport  Port=4
  wires:
  MATLAB Function/7(tack_count) -> Unit Delay/1
  Unit Delay2/1 -> MATLAB Function/14("prev_tacking ")
  GWP/1 -> MATLAB Function/1(target_WP)
  Unit Delay/1 -> MATLAB Function/15("tack_count ")
  MATLAB Function/6(prev_tacking) -> Unit Delay2/1
  Unit Delay3/1 -> MATLAB Function/13("typeC ")
  MATLAB Function/5(typeC) -> Unit Delay3/1
  MATLAB Function/1(chi_selected) -> Unit Delay1/1, chi_selected/1
  q/1 -> MATLAB Function/3(q)
  Constant1/1 -> MATLAB Function/6(beta_c)
  Constant10/1 -> MATLAB Function/8(beta_w)
  prev_GWP/1 -> MATLAB Function/2(prev_WP)
  chi/1 -> MATLAB Function/4(chi)
  Constant9/1 -> MATLAB Function/7(U_c)
  Constant13/1 -> MATLAB Function/11(tacking_plus)
  MATLAB Function/4(tacking) -> Terminator1/1  "Tacking on"
  Constant12/1 -> MATLAB Function/10(tacking_minus)
  Unit Delay1/1 -> MATLAB Function/16(prev_chi_selected)
  MATLAB Function/3(y__p_e) -> y__e_p/1
  MATLAB Function/9(prev_WP_original) -> Unit Delay4/1
  Unit Delay4/1 -> MATLAB Function/18("prev_WP_original ")
  MATLAB Function/8(prev_WP_update) -> Unit Delay5/1
  Unit Delay5/1 -> MATLAB Function/17("prev_WP_update ")
  MATLAB Function/10(ssa_on) -> Unit Delay6/1, ssa_on/1  "SSA on"
  Unit Delay6/1 -> MATLAB Function/19("ssa_on ")
  U_r/1 -> Selector/1
  Selector/1 -> MATLAB Function/5(U_rc)
  Constant2/1 -> MATLAB Function/12(delta)
  MATLAB Function/11(jib_angle) -> Unit Delay7/1
  Unit Delay7/1 -> MATLAB Function/20("jib_angle ")
  MATLAB Function/2(x__p_e) -> x__p_e/1
  U_w/1(Out1) -> MATLAB Function/9(U_w)

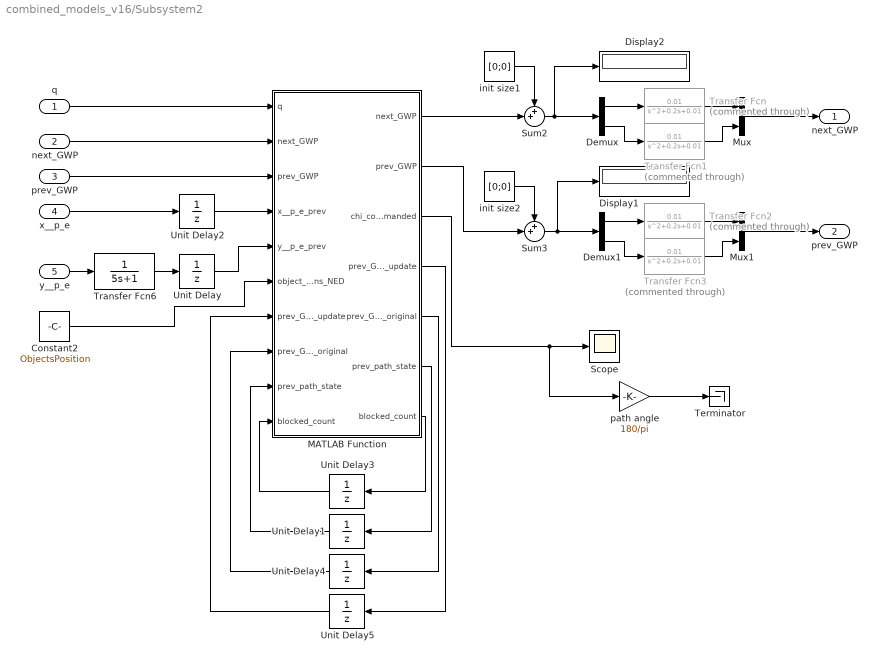
== system combined_models_v16/Subsystem2 ==
  q : Inport
  "next_GWP " : Inport  Port=2
  "prev_GWP " : Inport  Port=3
  x__p_e : Inport  Port=4
  y__p_e : Inport  Port=5
  Constant2 : Constant  Value=ObjectsPosition
  Demux : Demux  Outputs=2
  Demux1 : Demux  Outputs=2
  Display1 : Display
  Display2 : Display
  MATLAB Function : MATLAB Function  TreatAsAtomicUnit=on
  Mux : Mux  Inputs=2
  Mux1 : Mux  Inputs=2
  Scope : Scope
  Sum2 : Sum  Inputs=++|
  Sum3 : Sum  Inputs=++|
  Terminator : Terminator
  Transfer Fcn{,1..3} (4 alike) : TransferFcn  Commented=through  Numerator=[0.01]  Denominator=[1 0.2 0.01]
  Transfer Fcn6 : TransferFcn  Denominator=[5 1]
  Unit Delay{,1..3} (4 alike) : UnitDelay  SampleTime=-1  HasFrameUpgradeWarning=on
  Unit Delay4 : UnitDelay  InitialCondition=[0;0]  SampleTime=-1  HasFrameUpgradeWarning=on
  Unit Delay5 : UnitDelay  InitialCondition=NaN(2,1)  SampleTime=-1  HasFrameUpgradeWarning=on
  init size1 : Constant  Value=[0;0]
  init size2 : Constant  Value=[0;0]
  path angle : Gain  Gain=180/pi
  next_GWP : Outport
  prev_GWP : Outport  Port=2
  wires:
  Constant2/1 -> MATLAB Function/6(object_locations_NED)
  Unit Delay2/1 -> MATLAB Function/4(x__p_e_prev)
  "next_GWP "/1 -> MATLAB Function/2("next_GWP ")
  Unit Delay/1 -> MATLAB Function/5(y__p_e_prev)
  "prev_GWP "/1 -> MATLAB Function/3("prev_GWP ")
  q/1 -> MATLAB Function/1(q)
  x__p_e/1 -> Unit Delay2/1
  init size2/1 -> Sum3/1
  MATLAB Function/2(prev_GWP) -> Sum3/2
  Sum3/1 -> Demux1/1, Display1/1
  init size1/1 -> Sum2/1
  Sum2/1 -> Demux/1, Display2/1
  MATLAB Function/1(next_GWP) -> Sum2/2
  MATLAB Function/3(chi_commanded) -> path angle/1, Scope/1
  Mux/1 -> next_GWP/1
  Transfer Fcn/1 -> Mux/1
  Demux/1 -> Transfer Fcn/1
  Demux/2 -> Transfer Fcn1/1
  Transfer Fcn1/1 -> Mux/2
  Demux1/1 -> Transfer Fcn2/1
  Mux1/1 -> prev_GWP/1
  Transfer Fcn3/1 -> Mux1/2
  Demux1/2 -> Transfer Fcn3/1
  Transfer Fcn2/1 -> Mux1/1
  MATLAB Function/5(prev_GWP_original) -> Unit Delay4/1
  Unit Delay4/1 -> MATLAB Function/8("prev_GWP_original ")
  MATLAB Function/4(prev_GWP_update) -> Unit Delay5/1
  Unit Delay5/1 -> MATLAB Function/7("prev_GWP_update ")
  y__p_e/1 -> Transfer Fcn6/1
  Transfer Fcn6/1 -> Unit Delay/1
  MATLAB Function/6(prev_path_state) -> Unit Delay1/1
  Unit Delay1/1 -> MATLAB Function/9("prev_path_state ")
  MATLAB Function/7(blocked_count) -> Unit Delay3/1
  Unit Delay3/1 -> MATLAB Function/10("blocked_count ")
  path angle/1 -> Terminator/1

== system combined_models_v16/Velocity logger3 ==
  nu : Inport
  epsilon_dot and detla_t_dot : Inport  Port=2
  epsilon_dot_d : Inport  Port=3
  delta_t_dot_d : Inport  Port=4
  Demux1 : Demux  Outputs=3
  Demux4 : Demux  Outputs=2
  Demux5 : Demux  Outputs=3
  MATLAB Function1 : MATLAB Function  TreatAsAtomicUnit=on
  Mux : Mux  Inputs=2
  Mux10 : Mux  Inputs=2
  Mux9 : Mux  Inputs=2
  Scope1 : Scope  NumInputPorts=3
  Scope2 : Scope  NumInputPorts=3
  Scope4 : Scope  NumInputPorts=2
  Selector1 : Selector  InputPortWidth=8  IndexOptions=Index vector (dialog)  Indices=[1 2 4 6 7 8]  OutputSizes=1
  Selector7 : Selector  InputPortWidth=6  IndexOptions=Index vector (dialog)  Indices=[1 2 3]  OutputSizes=1
  Selector8 : Selector  InputPortWidth=6  IndexOptions=Index vector (dialog)  Indices=[4 5 6]  OutputSizes=1
  Terminator{,1,3..6} (6 alike) : Terminator
  To Workspace1 : ToWorkspace  VariableName=q_dot_state_lin  SampleTime=-1
  To Workspace2 : ToWorkspace  VariableName=q_dot_state_red_lin  SampleTime=simulation_sampling_time
  To Workspace3 : ToWorkspace  VariableName=crab_angle_si  SampleTime=simulation_sampling_time
  To Workspace4 : ToWorkspace  VariableName=speed_states_si  SampleTime=simulation_sampling_time
  q_dot_state_lin : Demux  Outputs=8
  wires:
  Selector8/1 -> Demux5/1
  Demux4/1 -> Mux9/1
  nu/1 -> Selector8/1, Selector7/1, Mux/1
  delta_t_dot_d/1 -> Mux10/2
  Demux4/2 -> Mux10/1
  epsilon_dot_d/1 -> Mux9/2
  epsilon_dot and detla_t_dot/1 -> Demux4/1, Mux/2
  Mux/1 -> To Workspace1/1, q_dot_state_lin/1, Selector1/1  "q_dot_state_lin"
  q_dot_state_lin/1 -> Scope1/1  "u"
  q_dot_state_lin/4 -> Scope2/1  "p"
  q_dot_state_lin/5 -> Scope2/2  "q"
  q_dot_state_lin/2 -> Scope1/2  "v"
  q_dot_state_lin/7 -> Scope4/1  "q_2"
  q_dot_state_lin/3 -> Scope1/3  "w"
  q_dot_state_lin/8 -> Scope4/2  "q_3"
  q_dot_state_lin/6 -> Scope2/3  "r"
  Selector1/1 -> To Workspace2/1
  Mux9/1 -> Terminator/1
  Mux10/1 -> Terminator1/1
  Demux5/1 -> Terminator3/1
  Demux5/2 -> Terminator4/1
  Demux5/3 -> Terminator5/1
  MATLAB Function1/2(beta_c) -> To Workspace3/1
  Demux1/3 -> Terminator6/1
  MATLAB Function1/1(U) -> To Workspace4/1
  Demux1/2 -> MATLAB Function1/2(v)
  Demux1/1 -> MATLAB Function1/1(u)
  Selector7/1 -> Demux1/1

== system combined_models_v16/WP Manager ==
  q : Inport
  WP : Inport  Port=2
  MATLAB Function1 : MATLAB Function  TreatAsAtomicUnit=on
  Rate Transition2 : RateTransition  OutPortSampleTime=WP_samplingtime
  Unit Delay : UnitDelay  InitialCondition=2  SampleTime=-1  HasFrameUpgradeWarning=on
  Unit Delay1 : UnitDelay  InitialCondition=1  SampleTime=-1  HasFrameUpgradeWarning=on
  Unit Delay2 : UnitDelay  InitialCondition=[0;0]  SampleTime=-1  HasFrameUpgradeWarning=on
  next_wp : Outport
  prev_wp : Outport  Port=2
  local path complete : Outport  Port=3
  wires:
  WP/1 -> MATLAB Function1/2(WP)
  Rate Transition2/1 -> MATLAB Function1/1(q)
  MATLAB Function1/2(next_wp) -> next_wp/1
  MATLAB Function1/4(next_wp_index) -> Unit Delay/1
  Unit Delay1/1 -> MATLAB Function1/4("prev_wp_index ")
  MATLAB Function1/3(prev_wp) -> prev_wp/1
  MATLAB Function1/5(prev_wp_index) -> Unit Delay1/1
  Unit Delay/1 -> MATLAB Function1/3("next_wp_index ")
  q/1 -> Rate Transition2/1
  MATLAB Function1/1(local_path_complete) -> local path complete/1
  MATLAB Function1/6(firstWP) -> Unit Delay2/1
  Unit Delay2/1 -> MATLAB Function1/5("firstWP ")

== system combined_models_v16/keel AOA controller ==
  note: With main velocity along the direction of travel, a positive AOA is achieved by
      | a negative change of the heading direction hence the invertion
  alpha_k_d : Inport
  AOAs : Inport  Port=2
  Gain : Gain  Gain=-1
  Saturation : Saturate  UpperLimit=15*pi/180  LowerLimit=-15*pi/180
  Selector1 : Selector  InputPortWidth=4  IndexOptions=Index vector (dialog)  Indices=[1]  OutputSizes=1
  Sum3 : Sum  Inputs=|+-
  psi_compensation : Outport
  wires:
  Selector1/1 -> Sum3/2  "alpha_k"
  Sum3/1 -> Gain/1  "alpha_k_error"
  AOAs/1 -> Selector1/1
  Gain/1 -> psi_compensation/1  "heading error"
  alpha_k_d/1 -> Saturation/1
  Saturation/1 -> Sum3/1  "alpha_k_d"

== system combined_models_v16/sail AOA control system ==
  q_dot : Inport
  reference : Inport  Port=2
  AOA : Inport  Port=3
  AC relative velocity : Inport  Port=4
  Gain : Gain  Gain=180/pi
  Gain scheduler1 : Subsystem
  "Gain scheduling, adaptive gain  sail AOA PID" : Subsystem
  Sail AOA reference model1 : Subsystem
  Terminator : Terminator
  Terminator7 : Terminator
  tail_reference : Gain  Gain=180/pi
  delta_t_d : Outport
  ref1 : Outport  Port=2
  wires:
  AOA/1 -> "Gain scheduling, adaptive gain  sail AOA PID"/2(AOA)
  reference/1 -> Sail AOA reference model1/1(reference)
  AC relative velocity/1 -> "Gain scheduling, adaptive gain  sail AOA PID"/4(AC_relative velocity), Gain scheduler1/1(AC relative velocity)
  Gain/1 -> Terminator/1  "sail AOA reference"
  "Gain scheduling, adaptive gain  sail AOA PID"/1(desired tail_angle) -> tail_reference/1, delta_t_d/1  "delta_t_d"
  Gain scheduler1/1(wn_ref_sAOA) -> Sail AOA reference model1/2(natraul_frequency)
  Gain scheduler1/2(zeta_ref_sAOA) -> Sail AOA reference model1/3(damping ratio)
  Sail AOA reference model1/1(x_d) -> Gain/1, "Gain scheduling, adaptive gain  sail AOA PID"/1(AOA_x_d)
  Sail AOA reference model1/2(ref) -> ref1/1
  q_dot/1 -> "Gain scheduling, adaptive gain  sail AOA PID"/3(q_dot)
  tail_reference/1 -> Terminator7/1

== system combined_models_v16/sailsystem dynamics2 ==
  delta_t : Inport
  v__n_rw : Inport  Port=2
  1st order tail dynamics : Subsystem
  Sailsystem dynamics : Subsystem
  Subsystem : Subsystem
  Sum : Sum  Inputs=|+-
  Terminator : Terminator
  Terminator1 : Terminator
  Terminator2 : Terminator
  delta_t0 : Constant  Value=q0(8)
  delta_t_sim : Gain  Gain=180/pi
  sail AOA sim : Gain  Gain=180/pi
  xi_dot : Scope
  beta_U_rw : Outport
  xi_lin1 : Outport  Port=2
  tau_sailsystem : Outport  Port=3
  wires:
  v__n_rw/1 -> Subsystem/3(v__n_rw), Sailsystem dynamics/2(v__n_rw)
  delta_t/1 -> 1st order tail dynamics/2(delta_t_d)
  Sailsystem dynamics/3(xi_dot) -> xi_dot/1
  Sailsystem dynamics/1(beta_U_rw) -> Subsystem/1(beta_U_r), Sum/1, beta_U_rw/1  "beta_U_r"
  Sailsystem dynamics/2(xi) -> Subsystem/2(xi_lin), Sum/2, xi_lin1/1  "xi_lin"
  Subsystem/1(tau_sailsystem) -> tau_sailsystem/1
  1st order tail dynamics/1(delta_t_dot) -> Terminator/1
  delta_t0/1 -> 1st order tail dynamics/1(delta_t0)
  Sum/1 -> sail AOA sim/1
  sail AOA sim/1 -> Terminator1/1
  1st order tail dynamics/2(delta_t) -> delta_t_sim/1, Sailsystem dynamics/1(delta_t)
  delta_t_sim/1 -> Terminator2/1

== system combined_models_v16/tail angle control system ==
  q : Inport
  delta_t_d : Inport  Port=2
  q_dot : Inport  Port=3
  AOA : Inport  Port=4
  AC_relative velocity : Inport  Port=5
  q_ddot : Inport  Port=6
  Demux1 : Demux  Outputs=3
  Scope2 : Scope  NumInputPorts=2
  Tail angle controller : Subsystem
  Tail angle reference model : Subsystem
  Terminator : Terminator
  Terminator1 : Terminator
  tail actuator moment : Outport
  delta_t_d1 : Outport  Port=2
  wires:
  Tail angle reference model/1(x_d) -> Demux1/1, Tail angle controller/1(delta_x_d)
  q_dot/1 -> Tail angle controller/3(q_dot)
  Tail angle controller/1(tail_moment) -> tail actuator moment/1  "tail actuator moment"
  AOA/1 -> Tail angle controller/5(AOA)
  Tail angle reference model/2(delta_t_d) -> delta_t_d1/1
  Demux1/1 -> Scope2/2  "delta_t_d"
  delta_t_d/1 -> Scope2/1, Tail angle reference model/1(reference)
  q_ddot/1 -> Tail angle controller/4(q_ddot)
  AC_relative velocity/1 -> Tail angle controller/6(AC_relative velocity)
  q/1 -> Tail angle controller/2(q)
  Demux1/2 -> Terminator/1
  Demux1/3 -> Terminator1/1

== system combined_models_v16/v_wind ==
  Constant4 : Constant  Value=v_wind_unit
  MATLAB Function3 : MATLAB Function  TreatAsAtomicUnit=on
  Step32 : Step  Time=start_w_trans  Before=U_w  After=U_w+U_w_step  SampleTime=0
  Transfer Fcn1 : TransferFcn  Denominator=[timeconstant_w 1]
  y : Outport
  wires:
  Transfer Fcn1/1 -> MATLAB Function3/1(a)
  Constant4/1 -> MATLAB Function3/2(b)
  Step32/1 -> Transfer Fcn1/1
  MATLAB Function3/1(y) -> y/1

== system combined_models_v16/Heading PD control system1/Gain scheduler1 ==
  note: discrete low
      | level controller
  velocity : Inport
  Constant3 : Constant  Value=omega_n_heading2
  MATLAB Function : MATLAB Function  TreatAsAtomicUnit=on
  Rate Transition5 : RateTransition  OutPortSampleTime=heading_controller_samplingtime
  Transfer Fcn : TransferFcn  Denominator=[1 1]
  wn_ref_sAOA : Outport
  zeta_ref_sAOA : Outport  Port=2
  wires:
  velocity/1 -> Rate Transition5/1  "sail AC velocity"
  Transfer Fcn/1 -> MATLAB Function/1(U_rc)
  Rate Transition5/1 -> Transfer Fcn/1
  MATLAB Function/2(zeta_ref_sAOA) -> zeta_ref_sAOA/1
  MATLAB Function/1(wn_ref_sAOA) -> wn_ref_sAOA/1
  Constant3/1 -> MATLAB Function/2(omega_n_s)

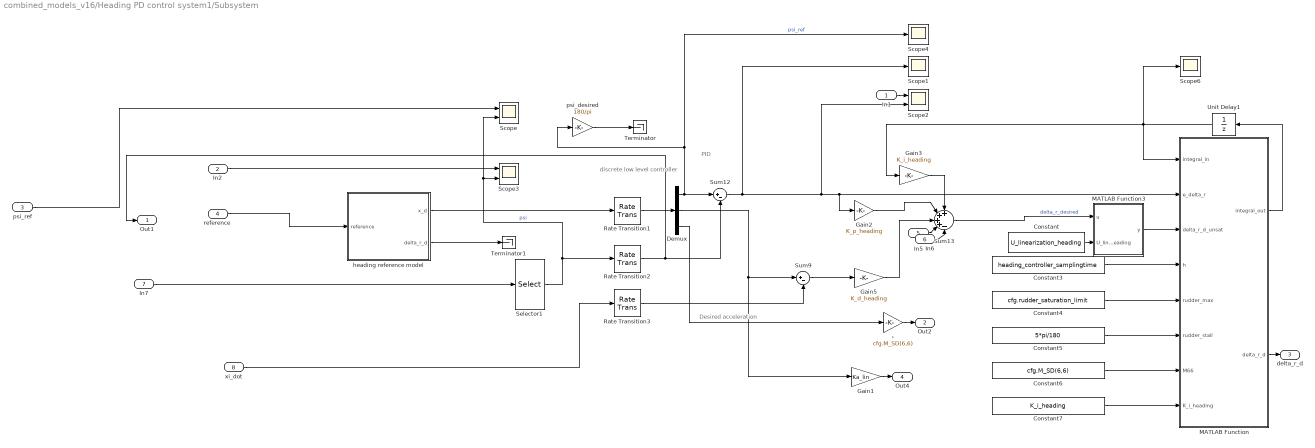
== system combined_models_v16/Heading PD control system1/Subsystem ==
  note: Desired acceleration
  note: PID
  note: discrete low
      | level controller
  In1 : Inport
  In2 : Inport  Port=2
  psi_ref : Inport  Port=3
  reference : Inport  Port=4
  In5 : Inport  Port=5
  In6 : Inport  Port=6
  In7 : Inport  Port=7
  xi_dot : Inport  Port=8
  - : Gain  Gain=cfg.M_SD(6,6)
  Constant : Constant  Value=U_linearization_heading
  Constant3 : Constant  Value=heading_controller_samplingtime
  Constant4 : Constant  Value=cfg.rudder_saturation_limit
  Constant5 : Constant  Value=5*pi/180
  Constant6 : Constant  Value=cfg.M_SD(6,6)
  Constant7 : Constant  Value=K_i_heading
  Demux : Demux  Outputs=3
  Gain1 : Gain  Gain=Ka_lin
  Gain2 : Gain  Gain=K_p_heading
  Gain3 : Gain  Gain=K_i_heading
  Gain5 : Gain  Gain=K_d_heading
  MATLAB Function : MATLAB Function  TreatAsAtomicUnit=on
  MATLAB Function3 : MATLAB Function  TreatAsAtomicUnit=on
  Rate Transition1 : RateTransition  OutPortSampleTime=heading_controller_samplingtime
  Rate Transition2 : RateTransition  OutPortSampleTime=heading_controller_samplingtime
  Rate Transition3 : RateTransition  OutPortSampleTime=heading_controller_samplingtime
  Scope : Scope  NumInputPorts=2
  Scope1 : Scope
  Scope2 : Scope  NumInputPorts=2
  Scope3 : Scope  NumInputPorts=2
  Scope4 : Scope
  Scope6 : Scope
  Selector1 : Selector  InputPortWidth=9  IndexOptions=Index vector (dialog)  Indices=[6]  OutputSizes=1
  Sum12 : Sum  Inputs=|+-
  Sum13 : Sum  Inputs=++++-
  Sum9 : Sum  Inputs=|+-
  Terminator : Terminator
  Terminator1 : Terminator
  Unit Delay1 : UnitDelay  SampleTime=-1  HasFrameUpgradeWarning=on
  heading reference model : Subsystem
  psi_desired : Gain  Gain=180/pi
  Out1 : Outport
  Out2 : Outport  Port=2
  delta_r_d : Outport  Port=3
  Out4 : Outport  Port=4
  wires:
  Constant6/1 -> MATLAB Function/7(M66)
  Sum13/1 -> MATLAB Function3/1(u)  "delta_r_desired"
  Selector1/1 -> Scope3/2, Scope/2, Rate Transition2/1  "psi"
  Constant4/1 -> MATLAB Function/5(rudder_max)
  Sum12/1 -> Scope2/2, Gain2/1, MATLAB Function/2(e_delta_r), Scope1/1
  reference/1 -> heading reference model/1(reference)
  Constant5/1 -> MATLAB Function/6(rudder_stall)
  MATLAB Function3/1(y) -> MATLAB Function/3(delta_r_d_unsat)
  Demux/1 -> Sum12/1, psi_desired/1, Scope4/1  "psi_ref"
  In5/1 -> Sum13/4
  heading reference model/2(delta_r_d) -> Terminator1/1
  Constant3/1 -> MATLAB Function/4(h)
  Demux/2 -> Gain1/1, Sum9/1
  MATLAB Function/2(delta_r_d) -> delta_r_d/1
  Constant7/1 -> MATLAB Function/8(K_i_heading)
  psi_ref/1 -> Scope/1
  heading reference model/1(x_d) -> Rate Transition1/1
  Demux/3 -> -/1
  In2/1 -> Scope3/1
  Rate Transition2/1 -> Out1/1, Sum12/2
  xi_dot/1 -> Rate Transition3/1
  Gain5/1 -> Sum13/3
  Gain3/1 -> Sum13/1
  Rate Transition1/1 -> Demux/1
  Gain2/1 -> Sum13/2
  In6/1 -> Sum13/5
  Sum9/1 -> Gain5/1
  Rate Transition3/1 -> Sum9/2
  Unit Delay1/1 -> Scope6/1, MATLAB Function/1(integral_in), Gain3/1
  Constant/1 -> MATLAB Function3/2(U_linearization_heading)
  MATLAB Function/1(integral_out) -> Unit Delay1/1
  psi_desired/1 -> Terminator/1
  Gain1/1 -> Out4/1
  In7/1 -> Selector1/1
  -/1 -> Out2/1
  In1/1 -> Scope2/1

== system combined_models_v16/Heading PD control system1/Subsystem1 ==
  note: PID
  In1 : Inport
  psi_ref : Inport  Port=2
  In3 : Inport  Port=3
  In4 : Inport  Port=4
  In5 : Inport  Port=5
  In6 : Inport  Port=6
  In7 : Inport  Port=7
  Constant2 : Constant  Commented=on  Value=U_linearization_heading
  Discrete-Time Integrator2 : DiscreteIntegrator  Commented=on  SampleTime=-1  ICPrevOutput=DiscIntNeverNeededParam  ICPrevScaledInput=DiscIntNeverNeededParam
  Gain6 : Gain  Commented=on  Gain=K_p_heading
  Gain7 : Gain  Commented=on  Gain=K_i_heading
  Gain8 : Gain  Commented=on  Gain=K_d_heading
  MATLAB Function1 : MATLAB Function  Commented=on  TreatAsAtomicUnit=on
  SSA++1 : MATLAB Function  Commented=on  TreatAsAtomicUnit=on
  SSA1 : MATLAB Function  Commented=on  TreatAsAtomicUnit=on
  Scope5 : Scope  Commented=on  NumInputPorts=2
  Sum1 : Sum  Commented=on  Inputs=|+-
  Sum2 : Sum  Commented=on  Inputs=+++
  Sum3 : Sum  Commented=on  Inputs=+--
  Sum4 : Sum  Commented=on  Inputs=|+-
  Out1 : Outport
  y : Outport  Port=2
  wires:
  SSA1/1(y) -> Scope5/2, Gain6/1, Gain7/1
  Gain7/1 -> Discrete-Time Integrator2/1
  Sum3/1 -> MATLAB Function1/1(u)  "delta_r_desired"
  Discrete-Time Integrator2/1 -> Sum2/1
  Constant2/1 -> MATLAB Function1/2(U_linearization_heading)
  MATLAB Function1/1(y) -> y/1
  Gain8/1 -> Sum2/3
  Gain6/1 -> Sum2/2
  Sum2/1 -> Sum3/1
  Sum4/1 -> Gain8/1
  Sum1/1 -> Out1/1, SSA1/1(error)
  In6/1 -> Sum4/1
  In7/1 -> Sum4/2
  In5/1 -> Sum1/2
  psi_ref/1 -> Sum1/1
  In1/1 -> Scope5/1
  In4/1 -> Sum3/3
  In3/1 -> Sum3/2

== system combined_models_v16/Heading PD control system1/heading reference model1 ==
  reference : Inport
  zeta_ref_heading : Inport  Port=2
  wn_ref_heading : Inport  Port=3
  Constant2 : Constant  Value=[theta0;0;0]
  Demux : Demux  Outputs=3
  Integrator : Integrator  InitialConditionSource=external
  MATLAB Function : MATLAB Function  TreatAsAtomicUnit=on
  Scope : Scope
  Scope1 : Scope
  Scope2 : Scope  NumInputPorts=2
  Terminator : Terminator
  Terminator1 : Terminator
  rate saturated ref model : Subsystem
  x_d : Outport
  delta_r_d : Outport  Port=2
  wires:
  MATLAB Function/1(x_refmod_dot) -> Integrator/1
  reference/1 -> rate saturated ref model/1(ref), Scope1/1, MATLAB Function/1(reference)
  Integrator/1 -> x_d/1, Scope/1, Scope2/2, MATLAB Function/4(x_refmod), Demux/1
  zeta_ref_heading/1 -> MATLAB Function/2(zeta_ref)
  wn_ref_heading/1 -> MATLAB Function/3(wn_ref)
  Constant2/1 -> Integrator/2
  Demux/2 -> Terminator/1
  Demux/3 -> Terminator1/1
  Demux/1 -> delta_r_d/1
  rate saturated ref model/1(desired) -> Scope2/1

== system combined_models_v16/Rudder dyanmics2/1st order rudder dynamics1 ==
  note: Create smooth saturation limits
  note: Positive rudder command
      | give positive heading angle
  note: Saturate angle input, so the derivative converge to 0 at saturation,
      | LP filter in order to maintain reasonable angular velocities
  delta_r0 : Inport
  delta_r_d : Inport  Port=2
  1/time constant : Gain  Gain=1/cfg.rudder_time_constant
  Integrator5 : Integrator  InitialConditionSource=external  InitialCondition=0.5
  Pos rudder give pos yaw : Gain  Gain=-1
  Saturation : Saturate  UpperLimit=cfg.rudder_saturation_limit  LowerLimit=-cfg.rudder_saturation_limit
  Saturation1 : Saturate  UpperLimit=cfg.rudder_saturation_limit  LowerLimit=-cfg.rudder_saturation_limit
  Sum6 : Sum  Inputs=|+-
  Transfer Fcn : TransferFcn  Denominator=[cfg.rudder_time_constant/10 1]
  Transfer Fcn1 : TransferFcn  Denominator=[cfg.rudder_time_constant/10 1]
  rudder gain : Gain  Gain=cfg.rudder_gain
  delta_r_dot : Outport
  delta_r : Outport  Port=2
  wires:
  Sum6/1 -> 1/time constant/1
  Integrator5/1 -> Saturation/1
  delta_r0/1 -> Integrator5/2
  delta_r_d/1 -> Pos rudder give pos yaw/1
  Saturation/1 -> Transfer Fcn/1
  Transfer Fcn/1 -> Sum6/2, delta_r/1
  Pos rudder give pos yaw/1 -> rudder gain/1
  1/time constant/1 -> delta_r_dot/1, Integrator5/1
  rudder gain/1 -> Saturation1/1
  Saturation1/1 -> Transfer Fcn1/1
  Transfer Fcn1/1 -> Sum6/1
